simulink model "ETS_Model"  (R2025a)
settings: Solver=FixedStepDiscrete  StartTime=0.0  StopTime=10.0  FixedStep=1e-5  RelTol=1e-3
libraries: spsSeriesRLCBranchLib x5, spsCurrentMeasurementLib x4, spsControlledVoltageSourceLib x3, spsDCVoltageSourceLib x1, simulink x1, spsUniversalBridgeLib x1, spsVoltageMeasurementLib x1, spspowerguiLib x1
settings Model: Creator=macbook  LastModifiedBy=macbook

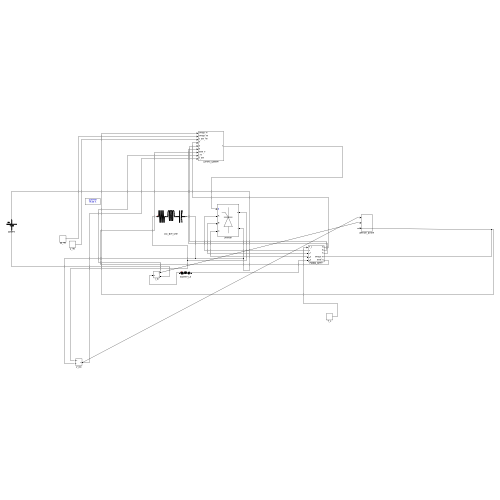
[thumbnail: Simulink's stored preview of the top-level diagram]
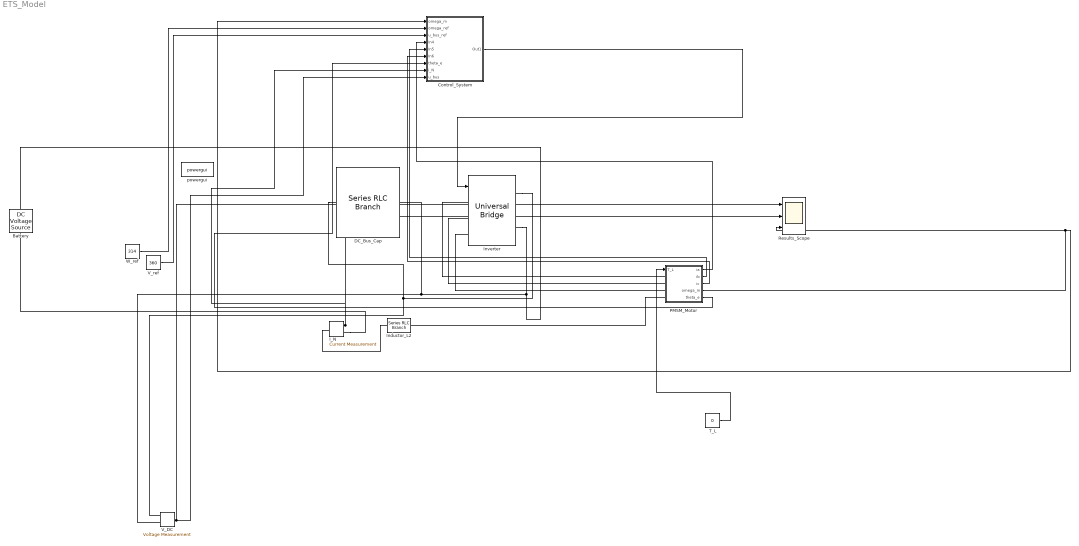
== system ETS_Model ==
  Battery : spsDCVoltageSourceLib/DC Voltage Source  Amplitude=100  Measurements=None
  Control_System : Subsystem
  DC_Bus_Cap : spsSeriesRLCBranchLib/Series RLC Branch  LConnTagsString=__new0  RConnTagsString=__new0  BranchType=RLC  Resistance=1  Inductance=1e-3  SetiL0=off  InitialCurrent=0  Capacitance=1e-6  Setx0=off  InitialVoltage=0  Measurements=None
  I_N : spsCurrentMeasurementLib/Current Measurement  PhasorSimulation=off  OutputType=Complex  PSBequivalent=0
  Inductor_L2 : spsSeriesRLCBranchLib/Series RLC Branch  LConnTagsString=__new0  RConnTagsString=__new0  BranchType=RLC  Resistance=1  Inductance=1e-3  SetiL0=off  InitialCurrent=0  Capacitance=1e-6  Setx0=off  InitialVoltage=0  Measurements=None
  Inverter : spsUniversalBridgeLib/Universal Bridge  Arms=3  SnubberResistance=1e5  SnubberCapacitance=inf  Device=Thyristors  Ron=1e-3  Lon=0  ForwardVoltages="[  0  0  ]"  ForwardVoltage=0  GTOparameters=[ 10e-6 , 20e-6 ]  IGBTparameters=[ 1e-6 , 2e-6 ]  Measurements=None  Measurements_2=None  converterType=Rectifier
  PMSM_Motor : Subsystem
  Results_Scope : Scope  NumInputPorts=3
  T_L : Constant  Value=0
  V_DC : spsVoltageMeasurementLib/Voltage Measurement  PhasorSimulation=off  OutputType=Complex  PSBequivalent=0
  V_ref : Constant  Value=360
  W_ref : Constant  Value=314
  powergui : spspowerguiLib/powergui  Priority=1  SimulationMode=Discrete  SampleTime=1e-5  frequency=60  Iterations=50  frequencyindice=0  Pbase=100e6  ErrMax=1e-4  UnitsV=kV  UnitsW=MW  buscounter=0  FunctionMessages=off  echomessages=off  EnableUseOfTLC=off  CurrentSourceSwitches=off  DisableSnubberDevices=off  DisableRonSwitches=off  DisableVfSwitches=off  DisplayEquations=off  AutomaticDiscreteSolvers=off  SolverType=Tustin/Backward Euler (TBE)  Interpol=off  ExternalGateDelay=off  methode=off  Ts=100  x0status=blocks  SPID=on  SwTol=0  HookPort=off  NonlinearTolerance=1e-4  nMaxIteration=100  ContinueOnMaxIteration=off  RestoreLinks=warning  ResistiveCurrentMeasurement=off  Frange=[0:2:500]  Ylog=off  Xlog=on  ShowGrid=off  save=off  variable=ZData  structure=0  ZoomFFT=off  StartTime=0.0  cycles=1  DisplayStyle=1  fundamental=60  FreqAxis=off  MaxFrequency=1000  frequencyindicesteady=1  RmsSteady=1  display=off
  wires:
  V_DC/1 -> Control_System/9(u_bus), Results_Scope/1
  I_N/1 -> Control_System/8(i_N), Results_Scope/2
  PMSM_Motor/4(omega_m) -> Control_System/1(omega_m), Results_Scope/3
  T_L/1 -> PMSM_Motor/1(T_L)
  W_ref/1 -> Control_System/2(omega_ref)
  V_ref/1 -> Control_System/3(u_bus_ref)
  PMSM_Motor/1(ia) -> Control_System/4(In4)
  PMSM_Motor/2(ib) -> Control_System/5(In5)
  PMSM_Motor/3(ic) -> Control_System/6(In6)
  PMSM_Motor/5(theta_e) -> Control_System/7(theta_e)
  Control_System/1(Out1) -> Inverter/1
  connections:
  DC_Bus_Cap/LConn1 -- V_DC/LConn1 -- Inverter/RConn1
  Inverter/RConn2 -- Battery/RConn1 -- DC_Bus_Cap/RConn1 -- V_DC/LConn2
  Inductor_L2/LConn1 -- I_N/LConn1
  I_N/RConn1 -- Battery/LConn1
  Inverter/LConn1 -- PMSM_Motor/LConn1
  Inverter/LConn2 -- PMSM_Motor/LConn2
  Inverter/LConn3 -- PMSM_Motor/LConn3
  PMSM_Motor/LConn4 -- Inductor_L2/RConn1

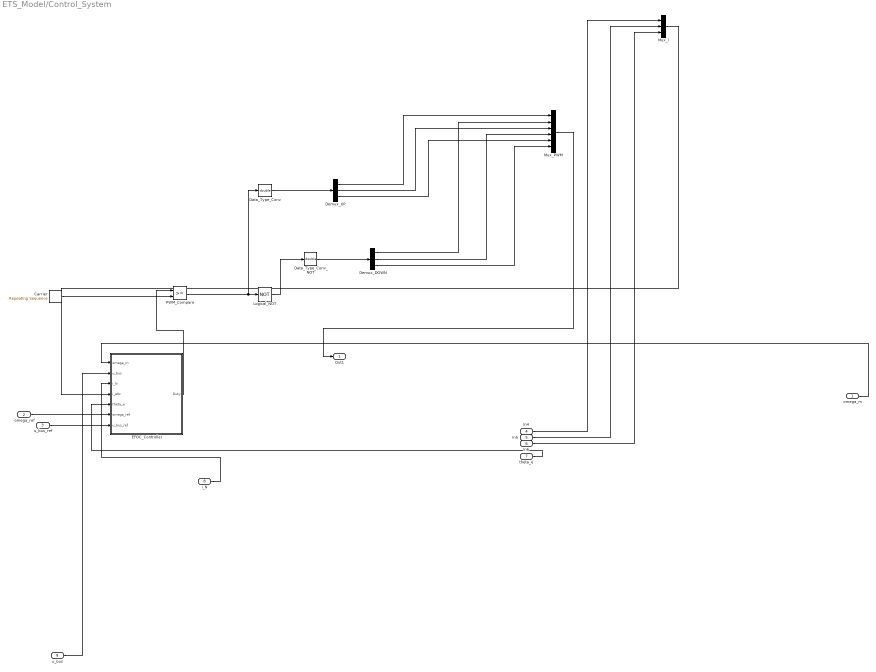
== system ETS_Model/Control_System ==
  omega_m : Inport
  omega_ref : Inport  Port=2
  u_bus_ref : Inport  Port=3
  In4 : Inport  Port=4
  In5 : Inport  Port=5
  In6 : Inport  Port=6
  theta_e : Inport  Port=7
  i_N : Inport  Port=8
  u_bus : Inport  Port=9
  Carrier : simulink/Sources/Repeating Sequence  rep_seq_t=[0 5e-5 1e-4]  rep_seq_y=[0 1 0]
  Data_Type_Conv : DataTypeConversion  OutDataTypeStr=double  SaturateOnIntegerOverflow=off  RndMeth=Floor
  Data_Type_Conv_NOT : DataTypeConversion  OutDataTypeStr=double  SaturateOnIntegerOverflow=off  RndMeth=Floor
  Demux_DOWN : Demux  Outputs=3
  Demux_UP : Demux  Outputs=3
  EFOC_Controller : MATLAB Function  TreatAsAtomicUnit=on
  Logical_NOT : Logic  Operator=NOT  AllPortsSameDT=off  OutDataTypeStr=boolean
  Mux_I : Mux  Inputs=3
  Mux_PWM : Mux  Inputs=6
  PWM_Compare : RelationalOperator  OutDataTypeStr=boolean  RndMeth=Simplest  InputSameDT=off
  Out1 : Outport
  wires:
  In6/1 -> Mux_I/3
  Demux_UP/1 -> Mux_PWM/1
  In5/1 -> Mux_I/2
  u_bus_ref/1 -> EFOC_Controller/7(u_bus_ref)
  In4/1 -> Mux_I/1
  Demux_UP/3 -> Mux_PWM/5
  theta_e/1 -> EFOC_Controller/5(theta_e)
  i_N/1 -> EFOC_Controller/3(i_N)
  omega_ref/1 -> EFOC_Controller/6(omega_ref)
  u_bus/1 -> EFOC_Controller/2(u_bus)
  omega_m/1 -> EFOC_Controller/1(omega_m)
  Demux_DOWN/1 -> Mux_PWM/2
  Carrier/1 -> PWM_Compare/2
  Demux_UP/2 -> Mux_PWM/3
  Mux_PWM/1 -> Out1/1
  Demux_DOWN/2 -> Mux_PWM/4
  Logical_NOT/1 -> Data_Type_Conv_NOT/1
  Mux_I/1 -> EFOC_Controller/4(i_abc)
  Data_Type_Conv/1 -> Demux_UP/1
  PWM_Compare/1 -> Data_Type_Conv/1, Logical_NOT/1
  Data_Type_Conv_NOT/1 -> Demux_DOWN/1
  Demux_DOWN/3 -> Mux_PWM/6
  EFOC_Controller/1(Duty) -> PWM_Compare/1

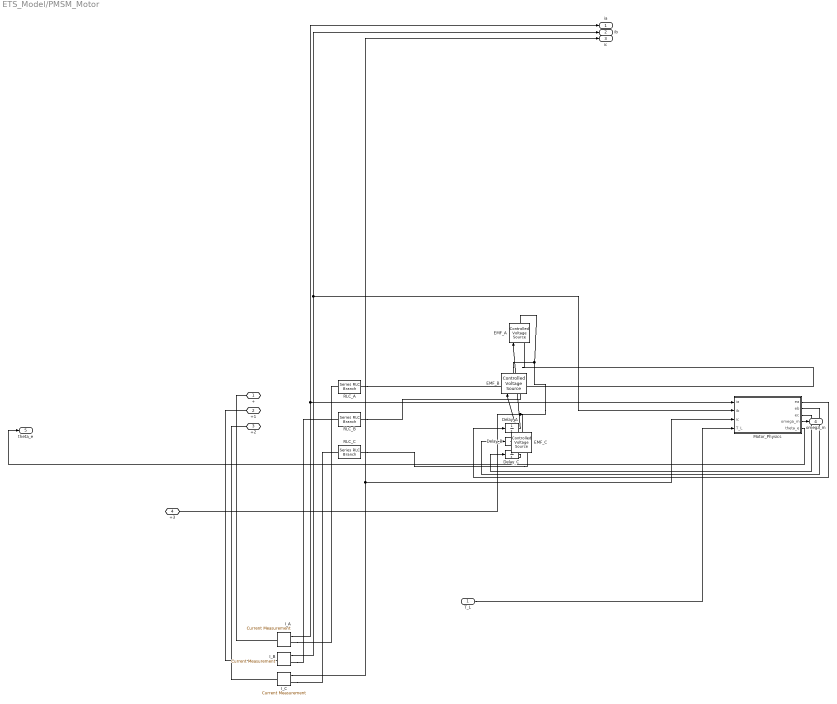
== system ETS_Model/PMSM_Motor ==
  T_L : Inport
  Delay_A : UnitDelay  SampleTime=1e-5  HasFrameUpgradeWarning=on
  Delay_B : UnitDelay  SampleTime=1e-5  HasFrameUpgradeWarning=on
  Delay_C : UnitDelay  SampleTime=1e-5  HasFrameUpgradeWarning=on
  EMF_A : spsControlledVoltageSourceLib/Controlled Voltage Source  Initialize=on  Source_Type=AC  Amplitude=0  Phase=0  Frequency=0  Measurements=None
  EMF_B : spsControlledVoltageSourceLib/Controlled Voltage Source  Initialize=on  Source_Type=AC  Amplitude=0  Phase=0  Frequency=0  Measurements=None
  EMF_C : spsControlledVoltageSourceLib/Controlled Voltage Source  Initialize=on  Source_Type=AC  Amplitude=0  Phase=0  Frequency=0  Measurements=None
  I_A : spsCurrentMeasurementLib/Current Measurement  PhasorSimulation=off  OutputType=Complex  PSBequivalent=0
  I_B : spsCurrentMeasurementLib/Current Measurement  PhasorSimulation=off  OutputType=Complex  PSBequivalent=0
  I_C : spsCurrentMeasurementLib/Current Measurement  PhasorSimulation=off  OutputType=Complex  PSBequivalent=0
  Motor_Physics : MATLAB Function  TreatAsAtomicUnit=on
  RLC_A : spsSeriesRLCBranchLib/Series RLC Branch  LConnTagsString=__new0  RConnTagsString=__new0  BranchType=RLC  Resistance=0.81  Inductance=1.5e-3  SetiL0=off  InitialCurrent=0  Capacitance=inf  Setx0=off  InitialVoltage=0  Measurements=None
  RLC_B : spsSeriesRLCBranchLib/Series RLC Branch  LConnTagsString=__new0  RConnTagsString=__new0  BranchType=RLC  Resistance=0.81  Inductance=1.5e-3  SetiL0=off  InitialCurrent=0  Capacitance=inf  Setx0=off  InitialVoltage=0  Measurements=None
  RLC_C : spsSeriesRLCBranchLib/Series RLC Branch  LConnTagsString=__new0  RConnTagsString=__new0  BranchType=RLC  Resistance=0.81  Inductance=1.5e-3  SetiL0=off  InitialCurrent=0  Capacitance=inf  Setx0=off  InitialVoltage=0  Measurements=None
  + : PMIOPort  Side=Left
  +1 : PMIOPort  Port=2  Side=Left
  +2 : PMIOPort  Port=3  Side=Left
  +3 : PMIOPort  Port=4  Side=Left
  ia : Outport
  ib : Outport  Port=2
  ic : Outport  Port=3
  omega_m : Outport  Port=4
  theta_e : Outport  Port=5
  wires:
  Motor_Physics/5(theta_e) -> theta_e/1
  Motor_Physics/4(omega_m) -> omega_m/1
  Motor_Physics/3(ec) -> Delay_C/1
  I_A/1 -> ia/1, Motor_Physics/1(ia)
  Delay_C/1 -> EMF_C/1
  Delay_A/1 -> EMF_A/1
  T_L/1 -> Motor_Physics/4(T_L)
  Delay_B/1 -> EMF_B/1
  Motor_Physics/2(eb) -> Delay_B/1
  Motor_Physics/1(ea) -> Delay_A/1
  I_B/1 -> ib/1, Motor_Physics/2(ib)
  I_C/1 -> ic/1, Motor_Physics/3(ic)
  connections:
  +2/RConn1 -- I_C/LConn1
  +1/RConn1 -- I_B/LConn1
  I_A/RConn1 -- RLC_A/LConn1
  EMF_B/RConn1 -- +3/RConn1 -- EMF_C/RConn1 -- EMF_A/RConn1
  RLC_A/RConn1 -- EMF_A/LConn1
  I_B/RConn1 -- RLC_B/LConn1
  RLC_C/RConn1 -- EMF_C/LConn1
  I_C/RConn1 -- RLC_C/LConn1
  +/RConn1 -- I_A/LConn1
  RLC_B/RConn1 -- EMF_B/LConn1

== matlab function ETS_Model/PMSM_Motor/Motor_Physics ==
  settings: updateMethod=DISCRETE
  data: ia input; ea output; ib input; ic input; T_L input; eb output; ec output; omega_m output; theta_e output
function [ea, eb, ec, omega_m, theta_e] = fcn(ia, ib, ic, T_L)
%#codegen
persistent w th
if isempty(w), w = 0; th = 0; end
Ts = 1e-5; p = 4; psi_f = 0.1; J = 0.005; B = 0.001; Ld = 1.5e-3; Lq = 1.5e-3;
ialpha = (2/3)*(ia - 0.5*ib - 0.5*ic);
ibeta = (2/3)*(sqrt(3)/2*ib - sqrt(3)/2*ic);
id = ialpha*cos(th) + ibeta*sin(th);
iq = -ialpha*sin(th) + ibeta*cos(th);
Te = 1.5 * p * (psi_f * iq + (Ld - Lq) * id * iq);
dw = (Te - T_L - B*w)/J;
w = w + dw*Ts;
th = th + w*p*Ts;
if th > 2*pi, th = th - 2*pi; end
if th < 0, th = th + 2*pi; end
omega_m = w; theta_e = th;
we = w*p;
ea = -we * psi_f * sin(th);
eb = -we * psi_f * sin(th - 2*pi/3);
ec = -we * psi_f * sin(th + 2*pi/3);

== matlab function ETS_Model/Control_System/EFOC_Controller ==
  data: omega_m input; Duty output; u_bus input; i_N input; i_abc input; theta_e input; omega_ref input; u_bus_ref input
function Duty = efoc_controller(omega_m, u_bus, i_N, i_abc, theta_e, omega_ref, u_bus_ref)
    %#codegen
    % Extended Field Oriented Control (EFOC) for Simulink MATLAB Function Block
    %
    % Inputs:
    % omega_m   : Mechanical speed (rad/s)
    % u_bus     : Measured DC bus voltage (V)
    % i_N       : Measured neutral point current (A)
    % i_abc     : 3-phase currents [i_a; i_b; i_c] (A)
    % theta_e   : Electrical angle (rad)
    % omega_ref : Reference mechanical speed (rad/s)
    % u_bus_ref : Reference DC bus voltage (e.g., 360 V)
    %
    % Outputs:
    % Duty      : PWM Duty cycles [D_a; D_b; D_c] (0.0 to 1.0)
    
    persistent int_id int_iq int_iN int_vbus int_spd
    if isempty(int_id)
        int_id = 0; int_iq = 0; int_iN = 0; int_vbus = 0; int_spd = 0;
    end
    
    Ts = 1e-4; % Controller sample time (10 kHz)
    
    % Hardcoded machine params (or pass via mask)
    p = 4; psi_f = 0.1; Ld = 1.5e-3; Lq = 1.5e-3; u_bat = 180;
    
    % Hardcoded PI gains (or pass via mask)
    Kp_id = 1.5; Ki_id = 810;
    Kp_iq = 1.5; Ki_iq = 810;
    Kp_iN = -0.016; Ki_iN = -0.75;
    Kp_vbus = 0.2; Ki_vbus = 5.0;
    Kp_spd = 0.1; Ki_spd = 2.0;
    
    %% 1. Park Transformation
    % Clarke
    i_alpha = (2/3) * (i_abc(1) - 0.5*i_abc(2) - 0.5*i_abc(3));
    i_beta = (2/3) * ((sqrt(3)/2)*i_abc(2) - (sqrt(3)/2)*i_abc(3));
    
    % Park
    id = i_alpha * cos(theta_e) + i_beta * sin(theta_e);
    iq = -i_alpha * sin(theta_e) + i_beta * cos(theta_e);
    
    %% 2. Speed Controller (PI)
    err_spd = omega_ref - omega_m;
    int_spd = int_spd + err_spd * Ts;
    int_spd = max(min(int_spd, 15), -15); % Anti-windup
    Te_ref = Kp_spd * err_spd + Ki_spd * int_spd;
    Te_ref = max(min(Te_ref, 15), -15);
    
    %% 3. MTPA (Surface PMSM -> id = 0)
    id_ref = 0;
    iq_ref = Te_ref / (1.5 * p * psi_f);
    
    %% 4. DC Bus Voltage Controller
    err_vbus = u_bus_ref - u_bus;
    int_vbus = int_vbus + err_vbus * Ts;
    int_vbus = max(min(int_vbus, 30), -30); % Anti-windup
    iN_ref = Kp_vbus * err_vbus + Ki_vbus * int_vbus;
    iN_ref = max(min(iN_ref, 30), -30);
    
    %% 5. Neutral Current Controller (Zero-Sequence DC/DC)
    err_iN = iN_ref - i_N;
    int_iN = int_iN + err_iN * Ts;
    
    % Feedforward term to decouple the battery voltage
    ff_D0 = u_bat / max(u_bus, 10.0); 
    D0 = ff_D0 + Kp_iN * err_iN + Ki_iN * int_iN;
    
    % Limit D0 to safe duty cycle boundaries
    if D0 > 0.9
        D0 = 0.9;
        int_iN = int_iN - err_iN * Ts; % Anti-windup
    elseif D0 < 0.1
        D0 = 0.1;
        int_iN = int_iN - err_iN * Ts;
    end
    
    %% 6. DQ Current Controllers
    err_id = id_ref - id;
    int_id = int_id + err_id * Ts;
    ud_star = Kp_id * err_id + Ki_id * int_id;
    
    err_iq = iq_ref - iq;
    int_iq = int_iq + err_iq * Ts;
    uq_star = Kp_iq * err_iq + Ki_iq * int_iq;
    
    % Cross-coupling decoupling
    omega_e = omega_m * p;
    ud_star = ud_star - omega_e * Lq * iq;
    uq_star = uq_star + omega_e * (psi_f + Ld * id);
    
    %% 7. Inverse Park Transformation
    u_alpha = ud_star * cos(theta_e) - uq_star * sin(theta_e);
    u_beta = ud_star * sin(theta_e) + uq_star * cos(theta_e);
    
    % Clarke Inverse
    u_AN_star = u_alpha;
    u_BN_star = -0.5 * u_alpha + (sqrt(3)/2) * u_beta;
    u_CN_star = -0.5 * u_alpha - (sqrt(3)/2) * u_beta;
    
    %% 8. Final Duty Cycle Generation (Eq 15)
    D_A = D0 + (u_AN_star / u_bus);
    D_B = D0 + (u_BN_star / u_bus);
    D_C = D0 + (u_CN_star / u_bus);
    
    % Saturate final duties
    Duty = [D_A; D_B; D_C];
    Duty = max(min(Duty, 1.0), 0.0);
end
